simulink model "FinalV2"  (R2018b)
settings: Solver=FixedStepAuto  StartTime=0.0  StopTime=1  RelTol=1e-3
values from neighbouring files (symbols this model uses):
  Kdi = dlqr(Ad,Bd,Q,R)    [finalScript.m]    (also in finalScriptV2.m)
  n = 16.5    [DC_motor_geared_integral_discrete_sysid23.m]    (also in DC_motor_geared_lqr_discrete_sysid23.m; finalScript.m; finalScriptV2.m)
  Tsc = 1/20000    (= 5e-05)    [DC_motor_geared_integral_discrete_sysid23.m]    (also in DC_motor_geared_lqr_discrete_sysid23.m = 1e-05; finalScript.m; finalScriptV2.m = 0.001)
undefined symbols (not defined in the file or in its folder): DiscIntNeverNeededParam
libraries: dspswit3 x29, mbedblockslib x19, simulink x10, dspsigops x5, powerlib_meascontrol x4, dspstat3 x2, peGeneralControl x1
(part 2 of 2)

== matlab function FinalV2/Snelheidsmeter Links/Periode meting ==
  data: speedPulse input; pulses output; speedPulseBuf data_store_memory; pulseCount data_store_memory; period input; i data_store_memory; fs input; j data_store_memory; reset input
function pulses = fcn(speedPulse,period, fs, reset)

global pulseCount;
global speedPulseBuf;
global i;
global j;

if reset == 1
    speedPulseBuf = uint8(zeros(size(speedPulseBuf)));
end

bufTime = period*fs + 1;

if i > bufTime
    i = uint32(1);
end

if j > bufTime
    j = uint32(1);
end

speedPulseBuf(i) = speedPulse;
pulseCount = pulseCount + uint32(speedPulse);
pulseCount = pulseCount - uint32(speedPulseBuf(j));

i = i + 1;
j = j + 1;

pulses = pulseCount;
